simulink model "exercise01"  (R2022a)
settings: Solver=VariableStepAuto  StartTime=0.0  StopTime=10.0  RelTol=1e-3
settings Model: Creator=cunis  LastModifiedBy=cunis

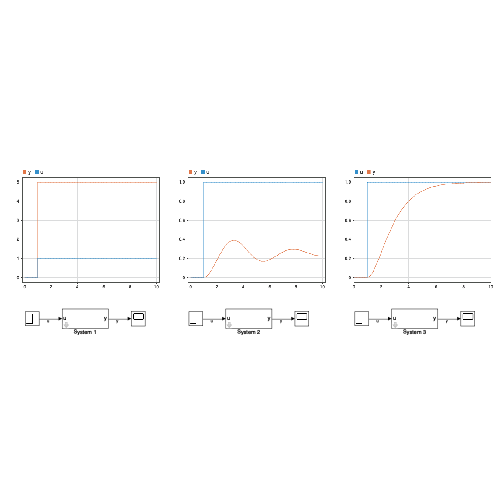
[thumbnail: Simulink's stored preview of the top-level diagram]
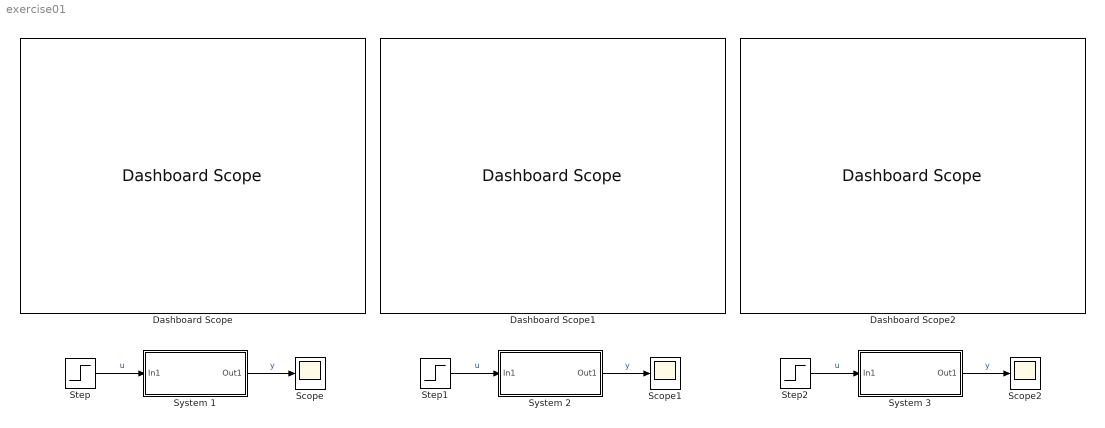
== system exercise01 ==
  Dashboard Scope : DashboardScope
  Dashboard Scope1 : DashboardScope
  Dashboard Scope2 : DashboardScope
  Scope : Scope
  Scope1 : Scope
  Scope2 : Scope
  Step : Step  SampleTime=0
  Step1 : Step  SampleTime=0
  Step2 : Step  SampleTime=0
  System 1 : Subsystem
      mask Display:
      | port_label('input',1,'u');
      | port_label('output',1,'y');
  System 2 : Subsystem
      mask Display:
      | port_label('input',1,'u');
      | port_label('output',1,'y');
  System 3 : Subsystem
      mask Display:
      | port_label('input',1,'u');
      | port_label('output',1,'y');
  wires:
  Step/1 -> System 1/1(In1)  "u"
  System 1/1(Out1) -> Scope/1  "y"
  System 2/1(Out1) -> Scope1/1  "y"
  Step1/1 -> System 2/1(In1)  "u"
  Step2/1 -> System 3/1(In1)  "u"
  System 3/1(Out1) -> Scope2/1  "y"

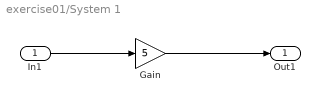
== system exercise01/System 1 ==
  In1 : Inport
  Gain : Gain  Gain=5
  Out1 : Outport
  wires:
  In1/1 -> Gain/1
  Gain/1 -> Out1/1

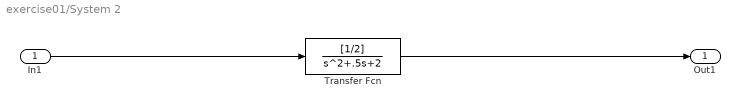
== system exercise01/System 2 ==
  In1 : Inport
  Transfer Fcn : TransferFcn  Numerator=[1/2]  Denominator=[1 .5 2]
  Out1 : Outport
  wires:
  In1/1 -> Transfer Fcn/1
  Transfer Fcn/1 -> Out1/1

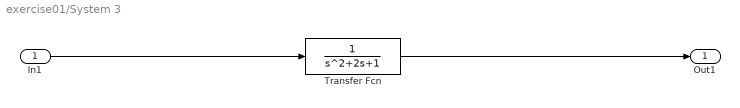
== system exercise01/System 3 ==
  In1 : Inport
  Transfer Fcn : TransferFcn
  Out1 : Outport
  wires:
  Transfer Fcn/1 -> Out1/1
  In1/1 -> Transfer Fcn/1
